simulink model "simulacao"  (R2018a)
settings: Solver=VariableStepAuto  StartTime=0.0  StopTime=10000  RelTol=1e-3
libraries: simulink x6
settings Model: Creator=Christopher  LastModifiedBy=Christopher

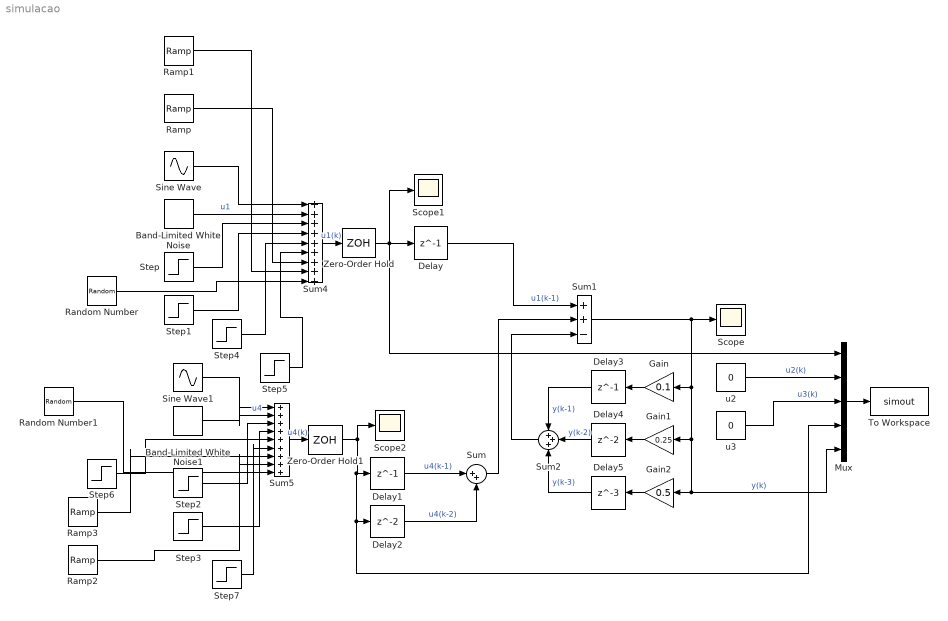
== system simulacao ==
  Band-Limited White Noise : simulink/Sources/Band-Limited White Noise  Cov=[0.005]  Ts=5  seed=[23341]
  Band-Limited White Noise1 : simulink/Sources/Band-Limited White Noise  Cov=[0.01]  Ts=5  seed=[333]
  Delay : Delay  DelayLength=1
  Delay1 : Delay  DelayLength=1
  Delay2 : Delay
  Delay3 : Delay  DelayLength=1
  Delay4 : Delay
  Delay5 : Delay  DelayLength=3
  Gain : Gain  Gain=0.1
  Gain1 : Gain  Gain=0.25
  Gain2 : Gain  Gain=0.5
  Mux : Mux  Inputs=5
  Ramp : simulink/Sources/Ramp  slope=0.0003  start=1000  InitialOutput=0
  Ramp1 : simulink/Sources/Ramp  slope=-0.0008  start=5000  InitialOutput=0
  Ramp2 : simulink/Sources/Ramp  slope=0.0005  start=2000  InitialOutput=0
  Ramp3 : simulink/Sources/Ramp  slope=-0.001  start=7000  InitialOutput=0
  Random Number : RandomNumber  Mean=1  Variance=0.005  Seed=25  SampleTime=250
  Random Number1 : RandomNumber  Mean=0.5  Variance=0.03  Seed=58  SampleTime=300
  Scope : Scope
  Scope1 : Scope
  Scope2 : Scope
  Sine Wave : Sin  SineType=Sample based  Amplitude=0.2  Samples=1000  SampleTime=1
  Sine Wave1 : Sin  SineType=Sample based  Amplitude=0.1  Samples=700  SampleTime=1  Offset=100
  Step : Step  Time=200  After=5  SampleTime=1
  Step1 : Step  Time=5000  After=5  SampleTime=1
  Step2 : Step  Time=3600  After=-2  SampleTime=1
  Step3 : Step  Time=8000  After=7  SampleTime=1
  Step4 : Step  Time=2000  After=10  SampleTime=1
  Step5 : Step  Time=8000  After=-3  SampleTime=1
  Step6 : Step  Time=100  After=3  SampleTime=1
  Step7 : Step  Time=5000  After=-1  SampleTime=1
  Sum : Sum  Inputs=|++
  Sum1 : Sum  Inputs=++-
  Sum2 : Sum  Inputs=+++
  Sum4 : Sum  Inputs=+++++++++
  Sum5 : Sum  Inputs=+++++++++
  To Workspace : ToWorkspace  VariableName=simout  SampleTime=-1
  Zero-Order Hold : ZeroOrderHold
  Zero-Order Hold1 : ZeroOrderHold
  u2 : Constant  Value=0  SampleTime=1
  u3 : Constant  Value=0  SampleTime=1
  wires:
  Delay1/1 -> Sum/1  "u4(k-1)"
  Delay2/1 -> Sum/2  "u4(k-2)"
  Delay/1 -> Sum1/1  "u1(k-1)"
  Sum/1 -> Sum1/2
  Sum1/1 -> Scope/1, Mux/5, Gain2/1, Gain1/1, Gain/1  "y(k)"
  Delay3/1 -> Sum2/1  "y(k-1)"
  Delay4/1 -> Sum2/2  "y(k-2)"
  Delay5/1 -> Sum2/3  "y(k-3)"
  Sum2/1 -> Sum1/3
  Mux/1 -> To Workspace/1
  u2/1 -> Mux/2  "u2(k)"
  u3/1 -> Mux/3  "u3(k)"
  Band-Limited White Noise/1 -> Sum4/2  "u1"
  Sum4/1 -> Zero-Order Hold/1  "u1(k)"
  Sine Wave/1 -> Sum4/1
  Step/1 -> Sum4/3
  Step1/1 -> Sum4/4
  Sum5/1 -> Zero-Order Hold1/1  "u4(k)"
  Band-Limited White Noise1/1 -> Sum5/2  "u4"
  Sine Wave1/1 -> Sum5/1
  Step2/1 -> Sum5/3
  Step3/1 -> Sum5/4
  Gain/1 -> Delay3/1
  Gain1/1 -> Delay4/1
  Gain2/1 -> Delay5/1
  Step4/1 -> Sum4/5
  Step5/1 -> Sum4/6
  Step6/1 -> Sum5/5
  Step7/1 -> Sum5/6
  Ramp/1 -> Sum4/7
  Ramp1/1 -> Sum4/8
  Ramp2/1 -> Sum5/8
  Ramp3/1 -> Sum5/7
  Random Number/1 -> Sum4/9
  Random Number1/1 -> Sum5/9
  Zero-Order Hold/1 -> Mux/1, Delay/1, Scope1/1
  Zero-Order Hold1/1 -> Scope2/1, Mux/4, Delay2/1, Delay1/1
